simulink model "aaa"  (R2016b)
settings: Solver=ode4  StartTime=0.0  StopTime=inf  FixedStep=0.002  RelTol=1e-3  EnableMultiTasking=on
libraries: slrtlib x3
(part 3 of 5)

== stateflow chart aaa/Subsystem1/zidong/1#3 ==
  state zidong
    state chushihua
      entry:
      skhx=0;
      kghx=0;
      kgzhiling1=0;
      kgzhiling2=0;
      yjhx=0;
      gghx=0;
      ggzhiling1=0;
      ggzhiling2=0;
      skt=0;
      kgt=0;
      sdt=0;
      jst=0;
      ggt=0;
      yjt=0;
      skyichang=0;
      kgyichang=0;
      sdyichang=0;
      jsyichang=0;
      ggyichang=0;
      yjyichang=0;
    state on1
      entry:
      skhx=1;
    state songkaishijian
      entry:
      skt=skt+0.002;
    state start
      entry:
      yikaicishu = 0;
    state on10
      entry:
      skyichang=1;
    state songkaishijian1
      entry:
      skt=skt+0.002;
    state on8
      entry:
      skhx=0;
    state yanchishijian1
      entry:
      t=t+1;
    state tguiling
      entry: t=0;
    state on2
      entry:
      skhx=0;
      kghx=1;
      kgzhiling1=1;
      kgzhiling2=1;
    state kaigaishijian
      entry:
      kgt=kgt+0.002;
    state stop
      entry:
      skhx=0;
      kghx=0;
      kgzhiling1=0;
      kgzhiling2=0;
      yjhx=0;
      gghx=0;
      ggzhiling1=0;
      ggzhiling2=0;
      skt=0;
      kgt=0;
      sdt=0;
      jst=0;
      ggt=0;
      yjt=0;
    state songkaishijian2
      entry:
      kgt=kgt+0.002;
    state on9
      entry:
      kghx=0;
      kgzhiling1=0;
      kgzhiling2=0;
    state on11
      entry:
      kgyichang=1;
    state yanchishijian2
      entry:
      t2=t2+1;
    state t2guiling
      entry: t2=0;
    state on3
      entry:
      kghx=0;
      kgzhiling1=0;
      kgzhiling2=0;
      yjhx=1;
    state suodingshijian
      entry:
      sdt=sdt+0.002;
    state on7
      entry:
      yikaicishu = yikaicishu + 1;
    state songkaishijian3
      entry:
      sdt=sdt+0.002;
    state on13
      entry:
      yjhx=0;
    state on12
      entry:
      sdyichang=1;
    state yanchishijian3
      entry:
      t4=t4+1;
    state t4guiling
      entry: t4=0;
    state off
      entry:
      skhx=0;
      kghx=0;
      kgzhiling1=0;
      kgzhiling2=0;
      yjhx=0;
      gghx=0;
      ggzhiling1=0;
      ggzhiling2=0;
      skt=0;
      kgt=0;
      sdt=0;
      jst=0;
      ggt=0;
      yjt=0;
    state on4
      entry:
      yjhx=0;
      skhx=1;
    state jiesuoshijian
      entry:
      jst=jst+0.002;
    state songkaishijian4
      entry:
      jst=jst+0.002;
    state on15
      entry:
      skhx=0;
    state on14
      entry:
      jsyichang=1;
    state yanchishijian4
      entry:
      t6=t6+1;
    state t6guiling
      entry: t6=0;
    state on5
      entry:
      skhx=0;
      gghx=1;
      ggzhiling1=1;
      ggzhiling2=1;
    state guangaishijian
      entry:
      ggt=ggt+0.002;
    state songkaishijian5
      entry:
      ggt=ggt+0.002;
    state on17
      entry:
      gghx=0;
      ggzhiling1=0;
      ggzhiling2=0;
    state on16
      entry:
      ggyichang=1;
    state yanchishijian5
      entry:
      t8=t8+1;
    state t8guiling
      entry: t8=0;
    state yanchishijian6
      entry:
      t10=t10+1;
    state t10guiling
      entry: t10=0;
    state on6
      entry:
      gghx=0;
      ggzhiling1=0;
      ggzhiling2=0;
      yjhx=1;
    state yajinshijian
      entry:
      yjt=yjt+0.002;
    state songkaishijian6
      entry:
      yjt=yjt+0.002;
    state on19
      entry:
      yjhx=0;
    state on18
      entry:
      ggyichang=1;
    (default) -> start
    songkaishijian1 -> songkaishijian1 [order 1] : [jsdw==0||skdw==0]
    chushihua -> on1 : [start==1&&ggdw1==1&&ggdw2==1&&yjdw==1&&sddw==1]
    on1 -> (junction 48)
    (junction 48) -> songkaishijian [order 1] : [jsdw==0||skdw==0]
    start -> chushihua : [start==1]
    (junction 348) -> (junction 48) [order 1] : [skt<=2]
    (junction 48) -> tguiling [order 2] : [jsdw==1&&skdw==1]
    songkaishijian -> (junction 348)
    songkaishijian1 -> on8 [order 2] : [jsdw==1&&skdw==1]
    on10 -> songkaishijian1
    (junction 348) -> on10 [order 2] : [skt>2]
    (junction 54) -> yanchishijian1 [order 1] : [t<t1]
    yanchishijian1 -> (junction 54) : after(500,tick)
    tguiling -> (junction 54)
    (junction 54) -> on2 [order 2] : [t>=t1]
    (junction 190) -> chushihua [order 1] : [yikaicishu<shedingcishu&&jieshu==0]
    songkaishijian2 -> songkaishijian2 [order 1] : [kgdw1==0||kgdw2==0||jsdw==0||skdw==0]
    on2 -> (junction 65)
    (junction 65) -> kaigaishijian [order 1] : [kgdw1==0||kgdw2==0||jsdw==0||skdw==0]
    (junction 361) -> (junction 65) [order 2] : [kgt<=12]
    (junction 65) -> t2guiling [order 2] : [kgdw1==1&&kgdw2==1&&jsdw==1&&skdw==1]
    kaigaishijian -> (junction 361)
    (junction 76) -> yanchishijian2 [order 1] : [t2<t3]
    songkaishijian2 -> on9 [order 2] : [kgdw1==1&&kgdw2==1&&jsdw==1&&skdw==1]
    on11 -> songkaishijian2
    (junction 361) -> on11 [order 1] : [kgt>12]
    (junction 190) -> stop [order 2] : [yikaicishu>=shedingcishu||jieshu==1]
    on7 -> (junction 190)
    yanchishijian2 -> (junction 76) : after(500,tick)
    t2guiling -> (junction 76)
    (junction 76) -> on3 [order 2] : [t2>=t3]
    songkaishijian3 -> songkaishijian3 [order 1] : [kgdw1==0||kgdw2==0||sddw==0||yjdw==0]
    on3 -> (junction 96)
    (junction 96) -> suodingshijian [order 1] : [kgdw1==0||kgdw2==0||sddw==0||yjdw==0]
    (junction 386) -> (junction 96) [order 2] : [sdt<=2]
    (junction 96) -> t4guiling [order 2] : [kgdw1==1&&kgdw2==1&&sddw==1&&yjdw==1]
    off -> on7
    suodingshijian -> (junction 386)
    (junction 105) -> yanchishijian3 [order 1] : [t4<t5]
    songkaishijian3 -> on13 [order 2] : [kgdw1==1&&kgdw2==1&&jsdw==1&&skdw==1]
    on12 -> songkaishijian3
    (junction 386) -> on12 [order 1] : [sdt>2]
    yanchishijian3 -> (junction 105) : after(500,tick)
    t4guiling -> (junction 105)
    (junction 105) -> on4 [order 2] : [t4>=t5]
    songkaishijian4 -> songkaishijian4 [order 1] : [kgdw1==0||kgdw2==0||jsdw==0||skdw==0]
    on4 -> (junction 115)
    (junction 115) -> jiesuoshijian [order 1] : [kgdw1==0||kgdw2==0||jsdw==0||skdw==0]
    (junction 390) -> (junction 115) [order 2] : [jst<=2]
    (junction 115) -> t6guiling [order 2] : [kgdw1==1&&kgdw2==1&&jsdw==1&&skdw==1]
    jiesuoshijian -> (junction 390)
    (junction 125) -> yanchishijian4 [order 1] : [t6<t7]
    songkaishijian4 -> on15 [order 2] : [kgdw1==1&&kgdw2==1&&jsdw==1&&skdw==1]
    on14 -> songkaishijian4
    (junction 390) -> on14 [order 1] : [jst>2]
    yanchishijian4 -> (junction 125) : after(500,tick)
    t6guiling -> (junction 125)
    (junction 125) -> on5 [order 2] : [t6>=t7]
    (junction 339) -> off [order 2] : [t10>=t11]
    songkaishijian5 -> songkaishijian5 [order 2] : [ggdw1==0||ggdw2==0||jsdw==0||skdw==0]
    on5 -> (junction 142)
    (junction 142) -> guangaishijian [order 1] : [ggdw1==0||ggdw2==0||jsdw==0||skdw==0]
    (junction 403) -> (junction 142) [order 2] : [ggt<=12]
    (junction 142) -> t8guiling [order 2] : [ggdw1==1&&ggdw2==1&&jsdw==1&&skdw==1]
    guangaishijian -> (junction 403)
    (junction 154) -> yanchishijian5 [order 1] : [t8<t9]
    songkaishijian5 -> on17 [order 1] : [ggdw1==1&&ggdw2==1&&jsdw==1&&skdw==1]
    on16 -> songkaishijian5
    (junction 403) -> on16 [order 1] : [ggt>12]
    yanchishijian5 -> (junction 154) : after(500,tick)
    t8guiling -> (junction 154)
    (junction 154) -> on6 [order 2] : [t8>=t9]
    yanchishijian6 -> (junction 339) : after(500,tick)
    (junction 339) -> yanchishijian6 [order 1] : [t10<t11]
    t10guiling -> (junction 339)
    (junction 162) -> t10guiling [order 2] : [sddw==1&&yjdw==1&&ggdw1==1&&ggdw2==1]
    on6 -> (junction 162)
    (junction 162) -> yajinshijian [order 1] : [sddw==0||yjdw==0]
    songkaishijian6 -> songkaishijian6 [order 2] : [sddw==0||yjdw==0]
    (junction 410) -> (junction 162) [order 2] : [yjt<=2]
    yajinshijian -> (junction 410)
    songkaishijian6 -> on19 [order 1] : [sddw==1&&yjdw==1&&ggdw1==1&&ggdw2==1]
    on18 -> songkaishijian6
    (junction 410) -> on18 [order 1] : [yjt>2]
  (default) -> zidong
  data: start input; kgdw1 input; kgdw2 input; skhx output; kghx output; kgzhiling1 output; kgzhiling2 output; yjhx output; gghx output; ggzhiling1 output; ggzhiling2 output; skt output; kgt output; sdt output; jst output; ggt output; yjt output; ggdw1 input; ggdw2 input; kghc input; gghc input; sddw input; yjdw input; skdw input; jsdw input; t1 input; t3 input; t5 input; t7 input; t9 input; t11 input; t local; t2 local; t4 local; t6 local; t8 local; shedingcishu input; yikaicishu output; skyichang output; kgyichang output; sdyichang output; jsyichang output; jieshu input; t10 local; ggyichang output; yjyichang output

== stateflow chart aaa/Subsystem1/zidong/1#4 ==
  state zidong
    state chushihua
      entry:
      skhx=0;
      kghx=0;
      kgzhiling1=0;
      kgzhiling2=0;
      yjhx=0;
      gghx=0;
      ggzhiling1=0;
      ggzhiling2=0;
      skt=0;
      kgt=0;
      sdt=0;
      jst=0;
      ggt=0;
      yjt=0;
      skyichang=0;
      kgyichang=0;
      sdyichang=0;
      jsyichang=0;
      ggyichang=0;
      yjyichang=0;
    state on1
      entry:
      skhx=1;
    state songkaishijian
      entry:
      skt=skt+0.002;
    state start
      entry:
      yikaicishu = 0;
    state on10
      entry:
      skyichang=1;
    state songkaishijian1
      entry:
      skt=skt+0.002;
    state on8
      entry:
      skhx=0;
    state yanchishijian1
      entry:
      t=t+1;
    state tguiling
      entry: t=0;
    state on2
      entry:
      skhx=0;
      kghx=1;
      kgzhiling1=1;
      kgzhiling2=1;
    state kaigaishijian
      entry:
      kgt=kgt+0.002;
    state stop
      entry:
      skhx=0;
      kghx=0;
      kgzhiling1=0;
      kgzhiling2=0;
      yjhx=0;
      gghx=0;
      ggzhiling1=0;
      ggzhiling2=0;
      skt=0;
      kgt=0;
      sdt=0;
      jst=0;
      ggt=0;
      yjt=0;
    state songkaishijian2
      entry:
      kgt=kgt+0.002;
    state on9
      entry:
      kghx=0;
      kgzhiling1=0;
      kgzhiling2=0;
    state on11
      entry:
      kgyichang=1;
    state yanchishijian2
      entry:
      t2=t2+1;
    state t2guiling
      entry: t2=0;
    state on3
      entry:
      kghx=0;
      kgzhiling1=0;
      kgzhiling2=0;
      yjhx=1;
    state suodingshijian
      entry:
      sdt=sdt+0.002;
    state on7
      entry:
      yikaicishu = yikaicishu + 1;
    state songkaishijian3
      entry:
      sdt=sdt+0.002;
    state on13
      entry:
      yjhx=0;
    state on12
      entry:
      sdyichang=1;
    state yanchishijian3
      entry:
      t4=t4+1;
    state t4guiling
      entry: t4=0;
    state off
      entry:
      skhx=0;
      kghx=0;
      kgzhiling1=0;
      kgzhiling2=0;
      yjhx=0;
      gghx=0;
      ggzhiling1=0;
      ggzhiling2=0;
      skt=0;
      kgt=0;
      sdt=0;
      jst=0;
      ggt=0;
      yjt=0;
    state on4
      entry:
      yjhx=0;
      skhx=1;
    state jiesuoshijian
      entry:
      jst=jst+0.002;
    state songkaishijian4
      entry:
      jst=jst+0.002;
    state on15
      entry:
      skhx=0;
    state on14
      entry:
      jsyichang=1;
    state yanchishijian4
      entry:
      t6=t6+1;
    state t6guiling
      entry: t6=0;
    state on5
      entry:
      skhx=0;
      gghx=1;
      ggzhiling1=1;
      ggzhiling2=1;
    state guangaishijian
      entry:
      ggt=ggt+0.002;
    state songkaishijian5
      entry:
      ggt=ggt+0.002;
    state on17
      entry:
      gghx=0;
      ggzhiling1=0;
      ggzhiling2=0;
    state on16
      entry:
      ggyichang=1;
    state yanchishijian5
      entry:
      t8=t8+1;
    state t8guiling
      entry: t8=0;
    state yanchishijian6
      entry:
      t10=t10+1;
    state t10guiling
      entry: t10=0;
    state on6
      entry:
      gghx=0;
      ggzhiling1=0;
      ggzhiling2=0;
      yjhx=1;
    state yajinshijian
      entry:
      yjt=yjt+0.002;
    state songkaishijian6
      entry:
      yjt=yjt+0.002;
    state on19
      entry:
      yjhx=0;
    state on18
      entry:
      ggyichang=1;
    (default) -> start
    songkaishijian1 -> songkaishijian1 [order 1] : [jsdw==0||skdw==0]
    chushihua -> on1 : [start==1&&ggdw1==1&&ggdw2==1&&yjdw==1&&sddw==1]
    on1 -> (junction 48)
    (junction 48) -> songkaishijian [order 1] : [jsdw==0||skdw==0]
    start -> chushihua : [start==1]
    (junction 348) -> (junction 48) [order 1] : [skt<=2]
    (junction 48) -> tguiling [order 2] : [jsdw==1&&skdw==1]
    songkaishijian -> (junction 348)
    songkaishijian1 -> on8 [order 2] : [jsdw==1&&skdw==1]
    on10 -> songkaishijian1
    (junction 348) -> on10 [order 2] : [skt>2]
    (junction 54) -> yanchishijian1 [order 1] : [t<t1]
    yanchishijian1 -> (junction 54) : after(500,tick)
    tguiling -> (junction 54)
    (junction 54) -> on2 [order 2] : [t>=t1]
    (junction 190) -> chushihua [order 1] : [yikaicishu<shedingcishu&&jieshu==0]
    songkaishijian2 -> songkaishijian2 [order 1] : [kgdw1==0||kgdw2==0||jsdw==0||skdw==0]
    on2 -> (junction 65)
    (junction 65) -> kaigaishijian [order 1] : [kgdw1==0||kgdw2==0||jsdw==0||skdw==0]
    (junction 361) -> (junction 65) [order 2] : [kgt<=12]
    (junction 65) -> t2guiling [order 2] : [kgdw1==1&&kgdw2==1&&jsdw==1&&skdw==1]
    kaigaishijian -> (junction 361)
    (junction 76) -> yanchishijian2 [order 1] : [t2<t3]
    songkaishijian2 -> on9 [order 2] : [kgdw1==1&&kgdw2==1&&jsdw==1&&skdw==1]
    on11 -> songkaishijian2
    (junction 361) -> on11 [order 1] : [kgt>12]
    (junction 190) -> stop [order 2] : [yikaicishu>=shedingcishu||jieshu==1]
    on7 -> (junction 190)
    yanchishijian2 -> (junction 76) : after(500,tick)
    t2guiling -> (junction 76)
    (junction 76) -> on3 [order 2] : [t2>=t3]
    songkaishijian3 -> songkaishijian3 [order 1] : [kgdw1==0||kgdw2==0||sddw==0||yjdw==0]
    on3 -> (junction 96)
    (junction 96) -> suodingshijian [order 1] : [kgdw1==0||kgdw2==0||sddw==0||yjdw==0]
    (junction 386) -> (junction 96) [order 2] : [sdt<=2]
    (junction 96) -> t4guiling [order 2] : [kgdw1==1&&kgdw2==1&&sddw==1&&yjdw==1]
    off -> on7
    suodingshijian -> (junction 386)
    (junction 105) -> yanchishijian3 [order 1] : [t4<t5]
    songkaishijian3 -> on13 [order 2] : [kgdw1==1&&kgdw2==1&&jsdw==1&&skdw==1]
    on12 -> songkaishijian3
    (junction 386) -> on12 [order 1] : [sdt>2]
    yanchishijian3 -> (junction 105) : after(500,tick)
    t4guiling -> (junction 105)
    (junction 105) -> on4 [order 2] : [t4>=t5]
    songkaishijian4 -> songkaishijian4 [order 1] : [kgdw1==0||kgdw2==0||jsdw==0||skdw==0]
    on4 -> (junction 115)
    (junction 115) -> jiesuoshijian [order 1] : [kgdw1==0||kgdw2==0||jsdw==0||skdw==0]
    (junction 390) -> (junction 115) [order 2] : [jst<=2]
    (junction 115) -> t6guiling [order 2] : [kgdw1==1&&kgdw2==1&&jsdw==1&&skdw==1]
    jiesuoshijian -> (junction 390)
    (junction 125) -> yanchishijian4 [order 1] : [t6<t7]
    songkaishijian4 -> on15 [order 2] : [kgdw1==1&&kgdw2==1&&jsdw==1&&skdw==1]
    on14 -> songkaishijian4
    (junction 390) -> on14 [order 1] : [jst>2]
    yanchishijian4 -> (junction 125) : after(500,tick)
    t6guiling -> (junction 125)
    (junction 125) -> on5 [order 2] : [t6>=t7]
    (junction 339) -> off [order 2] : [t10>=t11]
    songkaishijian5 -> songkaishijian5 [order 2] : [ggdw1==0||ggdw2==0||jsdw==0||skdw==0]
    on5 -> (junction 142)
    (junction 142) -> guangaishijian [order 1] : [ggdw1==0||ggdw2==0||jsdw==0||skdw==0]
    (junction 403) -> (junction 142) [order 2] : [ggt<=12]
    (junction 142) -> t8guiling [order 2] : [ggdw1==1&&ggdw2==1&&jsdw==1&&skdw==1]
    guangaishijian -> (junction 403)
    (junction 154) -> yanchishijian5 [order 1] : [t8<t9]
    songkaishijian5 -> on17 [order 1] : [ggdw1==1&&ggdw2==1&&jsdw==1&&skdw==1]
    on16 -> songkaishijian5
    (junction 403) -> on16 [order 1] : [ggt>12]
    yanchishijian5 -> (junction 154) : after(500,tick)
    t8guiling -> (junction 154)
    (junction 154) -> on6 [order 2] : [t8>=t9]
    yanchishijian6 -> (junction 339) : after(500,tick)
    (junction 339) -> yanchishijian6 [order 1] : [t10<t11]
    t10guiling -> (junction 339)
    (junction 162) -> t10guiling [order 2] : [sddw==1&&yjdw==1&&ggdw1==1&&ggdw2==1]
    on6 -> (junction 162)
    (junction 162) -> yajinshijian [order 1] : [sddw==0||yjdw==0]
    songkaishijian6 -> songkaishijian6 [order 2] : [sddw==0||yjdw==0]
    (junction 410) -> (junction 162) [order 2] : [yjt<=2]
    yajinshijian -> (junction 410)
    songkaishijian6 -> on19 [order 1] : [sddw==1&&yjdw==1&&ggdw1==1&&ggdw2==1]
    on18 -> songkaishijian6
    (junction 410) -> on18 [order 1] : [yjt>2]
  (default) -> zidong
  data: start input; kgdw1 input; kgdw2 input; skhx output; kghx output; kgzhiling1 output; kgzhiling2 output; yjhx output; gghx output; ggzhiling1 output; ggzhiling2 output; skt output; kgt output; sdt output; jst output; ggt output; yjt output; ggdw1 input; ggdw2 input; kghc input; gghc input; sddw input; yjdw input; skdw input; jsdw input; t1 input; t3 input; t5 input; t7 input; t9 input; t11 input; t local; t2 local; t4 local; t6 local; t8 local; shedingcishu input; yikaicishu output; skyichang output; kgyichang output; sdyichang output; jsyichang output; jieshu input; t10 local; ggyichang output; yjyichang output

== stateflow chart aaa/Subsystem1/zidong/1#5 ==
  state zidong
    state chushihua
      entry:
      skhx=0;
      kghx=0;
      kgzhiling1=0;
      kgzhiling2=0;
      yjhx=0;
      gghx=0;
      ggzhiling1=0;
      ggzhiling2=0;
      skt=0;
      kgt=0;
      sdt=0;
      jst=0;
      ggt=0;
      yjt=0;
      skyichang=0;
      kgyichang=0;
      sdyichang=0;
      jsyichang=0;
      ggyichang=0;
      yjyichang=0;
    state on1
      entry:
      skhx=1;
    state songkaishijian
      entry:
      skt=skt+0.002;
    state start
      entry:
      yikaicishu = 0;
    state on10
      entry:
      skyichang=1;
    state songkaishijian1
      entry:
      skt=skt+0.002;
    state on8
      entry:
      skhx=0;
    state yanchishijian1
      entry:
      t=t+1;
    state tguiling
      entry: t=0;
    state on2
      entry:
      skhx=0;
      kghx=1;
      kgzhiling1=1;
      kgzhiling2=1;
    state kaigaishijian
      entry:
      kgt=kgt+0.002;
    state stop
      entry:
      skhx=0;
      kghx=0;
      kgzhiling1=0;
      kgzhiling2=0;
      yjhx=0;
      gghx=0;
      ggzhiling1=0;
      ggzhiling2=0;
      skt=0;
      kgt=0;
      sdt=0;
      jst=0;
      ggt=0;
      yjt=0;
    state songkaishijian2
      entry:
      kgt=kgt+0.002;
    state on9
      entry:
      kghx=0;
      kgzhiling1=0;
      kgzhiling2=0;
    state on11
      entry:
      kgyichang=1;
    state yanchishijian2
      entry:
      t2=t2+1;
    state t2guiling
      entry: t2=0;
    state on3
      entry:
      kghx=0;
      kgzhiling1=0;
      kgzhiling2=0;
      yjhx=1;
    state suodingshijian
      entry:
      sdt=sdt+0.002;
    state on7
      entry:
      yikaicishu = yikaicishu + 1;
    state songkaishijian3
      entry:
      sdt=sdt+0.002;
    state on13
      entry:
      yjhx=0;
    state on12
      entry:
      sdyichang=1;
    state yanchishijian3
      entry:
      t4=t4+1;
    state t4guiling
      entry: t4=0;
    state off
      entry:
      skhx=0;
      kghx=0;
      kgzhiling1=0;
      kgzhiling2=0;
      yjhx=0;
      gghx=0;
      ggzhiling1=0;
      ggzhiling2=0;
      skt=0;
      kgt=0;
      sdt=0;
      jst=0;
      ggt=0;
      yjt=0;
    state on4
      entry:
      yjhx=0;
      skhx=1;
    state jiesuoshijian
      entry:
      jst=jst+0.002;
    state songkaishijian4
      entry:
      jst=jst+0.002;
    state on15
      entry:
      skhx=0;
    state on14
      entry:
      jsyichang=1;
    state yanchishijian4
      entry:
      t6=t6+1;
    state t6guiling
      entry: t6=0;
    state on5
      entry:
      skhx=0;
      gghx=1;
      ggzhiling1=1;
      ggzhiling2=1;
    state guangaishijian
      entry:
      ggt=ggt+0.002;
    state songkaishijian5
      entry:
      ggt=ggt+0.002;
    state on17
      entry:
      gghx=0;
      ggzhiling1=0;
      ggzhiling2=0;
    state on16
      entry:
      ggyichang=1;
    state yanchishijian5
      entry:
      t8=t8+1;
    state t8guiling
      entry: t8=0;
    state yanchishijian6
      entry:
      t10=t10+1;
    state t10guiling
      entry: t10=0;
    state on6
      entry:
      gghx=0;
      ggzhiling1=0;
      ggzhiling2=0;
      yjhx=1;
    state yajinshijian
      entry:
      yjt=yjt+0.002;
    state songkaishijian6
      entry:
      yjt=yjt+0.002;
    state on19
      entry:
      yjhx=0;
    state on18
      entry:
      ggyichang=1;
    (default) -> start
    songkaishijian1 -> songkaishijian1 [order 1] : [jsdw==0||skdw==0]
    chushihua -> on1 : [start==1&&ggdw1==1&&ggdw2==1&&yjdw==1&&sddw==1]
    on1 -> (junction 48)
    (junction 48) -> songkaishijian [order 1] : [jsdw==0||skdw==0]
    start -> chushihua : [start==1]
    (junction 348) -> (junction 48) [order 1] : [skt<=2]
    (junction 48) -> tguiling [order 2] : [jsdw==1&&skdw==1]
    songkaishijian -> (junction 348)
    songkaishijian1 -> on8 [order 2] : [jsdw==1&&skdw==1]
    on10 -> songkaishijian1
    (junction 348) -> on10 [order 2] : [skt>2]
    (junction 54) -> yanchishijian1 [order 1] : [t<t1]
    yanchishijian1 -> (junction 54) : after(500,tick)
    tguiling -> (junction 54)
    (junction 54) -> on2 [order 2] : [t>=t1]
    (junction 190) -> chushihua [order 1] : [yikaicishu<shedingcishu&&jieshu==0]
    songkaishijian2 -> songkaishijian2 [order 1] : [kgdw1==0||kgdw2==0||jsdw==0||skdw==0]
    on2 -> (junction 65)
    (junction 65) -> kaigaishijian [order 1] : [kgdw1==0||kgdw2==0||jsdw==0||skdw==0]
    (junction 361) -> (junction 65) [order 2] : [kgt<=12]
    (junction 65) -> t2guiling [order 2] : [kgdw1==1&&kgdw2==1&&jsdw==1&&skdw==1]
    kaigaishijian -> (junction 361)
    (junction 76) -> yanchishijian2 [order 1] : [t2<t3]
    songkaishijian2 -> on9 [order 2] : [kgdw1==1&&kgdw2==1&&jsdw==1&&skdw==1]
    on11 -> songkaishijian2
    (junction 361) -> on11 [order 1] : [kgt>12]
    (junction 190) -> stop [order 2] : [yikaicishu>=shedingcishu||jieshu==1]
    on7 -> (junction 190)
    yanchishijian2 -> (junction 76) : after(500,tick)
    t2guiling -> (junction 76)
    (junction 76) -> on3 [order 2] : [t2>=t3]
    songkaishijian3 -> songkaishijian3 [order 1] : [kgdw1==0||kgdw2==0||sddw==0||yjdw==0]
    on3 -> (junction 96)
    (junction 96) -> suodingshijian [order 1] : [kgdw1==0||kgdw2==0||sddw==0||yjdw==0]
    (junction 386) -> (junction 96) [order 2] : [sdt<=2]
    (junction 96) -> t4guiling [order 2] : [kgdw1==1&&kgdw2==1&&sddw==1&&yjdw==1]
    off -> on7
    suodingshijian -> (junction 386)
    (junction 105) -> yanchishijian3 [order 1] : [t4<t5]
    songkaishijian3 -> on13 [order 2] : [kgdw1==1&&kgdw2==1&&jsdw==1&&skdw==1]
    on12 -> songkaishijian3
    (junction 386) -> on12 [order 1] : [sdt>2]
    yanchishijian3 -> (junction 105) : after(500,tick)
    t4guiling -> (junction 105)
    (junction 105) -> on4 [order 2] : [t4>=t5]
    songkaishijian4 -> songkaishijian4 [order 1] : [kgdw1==0||kgdw2==0||jsdw==0||skdw==0]
    on4 -> (junction 115)
    (junction 115) -> jiesuoshijian [order 1] : [kgdw1==0||kgdw2==0||jsdw==0||skdw==0]
    (junction 390) -> (junction 115) [order 2] : [jst<=2]
    (junction 115) -> t6guiling [order 2] : [kgdw1==1&&kgdw2==1&&jsdw==1&&skdw==1]
    jiesuoshijian -> (junction 390)
    (junction 125) -> yanchishijian4 [order 1] : [t6<t7]
    songkaishijian4 -> on15 [order 2] : [kgdw1==1&&kgdw2==1&&jsdw==1&&skdw==1]
    on14 -> songkaishijian4
    (junction 390) -> on14 [order 1] : [jst>2]
    yanchishijian4 -> (junction 125) : after(500,tick)
    t6guiling -> (junction 125)
    (junction 125) -> on5 [order 2] : [t6>=t7]
    (junction 339) -> off [order 2] : [t10>=t11]
    songkaishijian5 -> songkaishijian5 [order 2] : [ggdw1==0||ggdw2==0||jsdw==0||skdw==0]
    on5 -> (junction 142)
    (junction 142) -> guangaishijian [order 1] : [ggdw1==0||ggdw2==0||jsdw==0||skdw==0]
    (junction 403) -> (junction 142) [order 2] : [ggt<=12]
    (junction 142) -> t8guiling [order 2] : [ggdw1==1&&ggdw2==1&&jsdw==1&&skdw==1]
    guangaishijian -> (junction 403)
    (junction 154) -> yanchishijian5 [order 1] : [t8<t9]
    songkaishijian5 -> on17 [order 1] : [ggdw1==1&&ggdw2==1&&jsdw==1&&skdw==1]
    on16 -> songkaishijian5
    (junction 403) -> on16 [order 1] : [ggt>12]
    yanchishijian5 -> (junction 154) : after(500,tick)
    t8guiling -> (junction 154)
    (junction 154) -> on6 [order 2] : [t8>=t9]
    yanchishijian6 -> (junction 339) : after(500,tick)
    (junction 339) -> yanchishijian6 [order 1] : [t10<t11]
    t10guiling -> (junction 339)
    (junction 162) -> t10guiling [order 2] : [sddw==1&&yjdw==1&&ggdw1==1&&ggdw2==1]
    on6 -> (junction 162)
    (junction 162) -> yajinshijian [order 1] : [sddw==0||yjdw==0]
    songkaishijian6 -> songkaishijian6 [order 2] : [sddw==0||yjdw==0]
    (junction 410) -> (junction 162) [order 2] : [yjt<=2]
    yajinshijian -> (junction 410)
    songkaishijian6 -> on19 [order 1] : [sddw==1&&yjdw==1&&ggdw1==1&&ggdw2==1]
    on18 -> songkaishijian6
    (junction 410) -> on18 [order 1] : [yjt>2]
  (default) -> zidong
  data: start input; kgdw1 input; kgdw2 input; skhx output; kghx output; kgzhiling1 output; kgzhiling2 output; yjhx output; gghx output; ggzhiling1 output; ggzhiling2 output; skt output; kgt output; sdt output; jst output; ggt output; yjt output; ggdw1 input; ggdw2 input; kghc input; gghc input; sddw input; yjdw input; skdw input; jsdw input; t1 input; t3 input; t5 input; t7 input; t9 input; t11 input; t local; t2 local; t4 local; t6 local; t8 local; shedingcishu input; yikaicishu output; skyichang output; kgyichang output; sdyichang output; jsyichang output; jieshu input; t10 local; ggyichang output; yjyichang output

== stateflow chart aaa/Subsystem1/zidong/1#6 ==
  state zidong
    state chushihua
      entry:
      skhx=0;
      kghx=0;
      kgzhiling1=0;
      kgzhiling2=0;
      yjhx=0;
      gghx=0;
      ggzhiling1=0;
      ggzhiling2=0;
      skt=0;
      kgt=0;
      sdt=0;
      jst=0;
      ggt=0;
      yjt=0;
      skyichang=0;
      kgyichang=0;
      sdyichang=0;
      jsyichang=0;
      ggyichang=0;
      yjyichang=0;
    state on1
      entry:
      skhx=1;
    state songkaishijian
      entry:
      skt=skt+0.002;
    state start
      entry:
      yikaicishu = 0;
    state on10
      entry:
      skyichang=1;
    state songkaishijian1
      entry:
      skt=skt+0.002;
    state on8
      entry:
      skhx=0;
    state yanchishijian1
      entry:
      t=t+1;
    state tguiling
      entry: t=0;
    state on2
      entry:
      skhx=0;
      kghx=1;
      kgzhiling1=1;
      kgzhiling2=1;
    state kaigaishijian
      entry:
      kgt=kgt+0.002;
    state stop
      entry:
      skhx=0;
      kghx=0;
      kgzhiling1=0;
      kgzhiling2=0;
      yjhx=0;
      gghx=0;
      ggzhiling1=0;
      ggzhiling2=0;
      skt=0;
      kgt=0;
      sdt=0;
      jst=0;
      ggt=0;
      yjt=0;
    state songkaishijian2
      entry:
      kgt=kgt+0.002;
    state on9
      entry:
      kghx=0;
      kgzhiling1=0;
      kgzhiling2=0;
    state on11
      entry:
      kgyichang=1;
    state yanchishijian2
      entry:
      t2=t2+1;
    state t2guiling
      entry: t2=0;
    state on3
      entry:
      kghx=0;
      kgzhiling1=0;
      kgzhiling2=0;
      yjhx=1;
    state suodingshijian
      entry:
      sdt=sdt+0.002;
    state on7
      entry:
      yikaicishu = yikaicishu + 1;
    state songkaishijian3
      entry:
      sdt=sdt+0.002;
    state on13
      entry:
      yjhx=0;
    state on12
      entry:
      sdyichang=1;
    state yanchishijian3
      entry:
      t4=t4+1;
    state t4guiling
      entry: t4=0;
    state off
      entry:
      skhx=0;
      kghx=0;
      kgzhiling1=0;
      kgzhiling2=0;
      yjhx=0;
      gghx=0;
      ggzhiling1=0;
      ggzhiling2=0;
      skt=0;
      kgt=0;
      sdt=0;
      jst=0;
      ggt=0;
      yjt=0;
    state on4
      entry:
      yjhx=0;
      skhx=1;
    state jiesuoshijian
      entry:
      jst=jst+0.002;
    state songkaishijian4
      entry:
      jst=jst+0.002;
    state on15
      entry:
      skhx=0;
    state on14
      entry:
      jsyichang=1;
    state yanchishijian4
      entry:
      t6=t6+1;
    state t6guiling
      entry: t6=0;
    state on5
      entry:
      skhx=0;
      gghx=1;
      ggzhiling1=1;
      ggzhiling2=1;
    state guangaishijian
      entry:
      ggt=ggt+0.002;
    state songkaishijian5
      entry:
      ggt=ggt+0.002;
    state on17
      entry:
      gghx=0;
      ggzhiling1=0;
      ggzhiling2=0;
    state on16
      entry:
      ggyichang=1;
    state yanchishijian5
      entry:
      t8=t8+1;
    state t8guiling
      entry: t8=0;
    state yanchishijian6
      entry:
      t10=t10+1;
    state t10guiling
      entry: t10=0;
    state on6
      entry:
      gghx=0;
      ggzhiling1=0;
      ggzhiling2=0;
      yjhx=1;
    state yajinshijian
      entry:
      yjt=yjt+0.002;
    state songkaishijian6
      entry:
      yjt=yjt+0.002;
    state on19
      entry:
      yjhx=0;
    state on18
      entry:
      ggyichang=1;
    (default) -> start
    songkaishijian1 -> songkaishijian1 [order 1] : [jsdw==0||skdw==0]
    chushihua -> on1 : [start==1&&ggdw1==1&&ggdw2==1&&yjdw==1&&sddw==1]
    on1 -> (junction 48)
    (junction 48) -> songkaishijian [order 1] : [jsdw==0||skdw==0]
    start -> chushihua : [start==1]
    (junction 348) -> (junction 48) [order 1] : [skt<=2]
    (junction 48) -> tguiling [order 2] : [jsdw==1&&skdw==1]
    songkaishijian -> (junction 348)
    songkaishijian1 -> on8 [order 2] : [jsdw==1&&skdw==1]
    on10 -> songkaishijian1
    (junction 348) -> on10 [order 2] : [skt>2]
    (junction 54) -> yanchishijian1 [order 1] : [t<t1]
    yanchishijian1 -> (junction 54) : after(500,tick)
    tguiling -> (junction 54)
    (junction 54) -> on2 [order 2] : [t>=t1]
    (junction 190) -> chushihua [order 1] : [yikaicishu<shedingcishu&&jieshu==0]
    songkaishijian2 -> songkaishijian2 [order 1] : [kgdw1==0||kgdw2==0||jsdw==0||skdw==0]
    on2 -> (junction 65)
    (junction 65) -> kaigaishijian [order 1] : [kgdw1==0||kgdw2==0||jsdw==0||skdw==0]
    (junction 361) -> (junction 65) [order 2] : [kgt<=12]
    (junction 65) -> t2guiling [order 2] : [kgdw1==1&&kgdw2==1&&jsdw==1&&skdw==1]
    kaigaishijian -> (junction 361)
    (junction 76) -> yanchishijian2 [order 1] : [t2<t3]
    songkaishijian2 -> on9 [order 2] : [kgdw1==1&&kgdw2==1&&jsdw==1&&skdw==1]
    on11 -> songkaishijian2
    (junction 361) -> on11 [order 1] : [kgt>12]
    (junction 190) -> stop [order 2] : [yikaicishu>=shedingcishu||jieshu==1]
    on7 -> (junction 190)
    yanchishijian2 -> (junction 76) : after(500,tick)
    t2guiling -> (junction 76)
    (junction 76) -> on3 [order 2] : [t2>=t3]
    songkaishijian3 -> songkaishijian3 [order 1] : [kgdw1==0||kgdw2==0||sddw==0||yjdw==0]
    on3 -> (junction 96)
    (junction 96) -> suodingshijian [order 1] : [kgdw1==0||kgdw2==0||sddw==0||yjdw==0]
    (junction 386) -> (junction 96) [order 2] : [sdt<=2]
    (junction 96) -> t4guiling [order 2] : [kgdw1==1&&kgdw2==1&&sddw==1&&yjdw==1]
    off -> on7
    suodingshijian -> (junction 386)
    (junction 105) -> yanchishijian3 [order 1] : [t4<t5]
    songkaishijian3 -> on13 [order 2] : [kgdw1==1&&kgdw2==1&&jsdw==1&&skdw==1]
    on12 -> songkaishijian3
    (junction 386) -> on12 [order 1] : [sdt>2]
    yanchishijian3 -> (junction 105) : after(500,tick)
    t4guiling -> (junction 105)
    (junction 105) -> on4 [order 2] : [t4>=t5]
    songkaishijian4 -> songkaishijian4 [order 1] : [kgdw1==0||kgdw2==0||jsdw==0||skdw==0]
    on4 -> (junction 115)
    (junction 115) -> jiesuoshijian [order 1] : [kgdw1==0||kgdw2==0||jsdw==0||skdw==0]
    (junction 390) -> (junction 115) [order 2] : [jst<=2]
    (junction 115) -> t6guiling [order 2] : [kgdw1==1&&kgdw2==1&&jsdw==1&&skdw==1]
    jiesuoshijian -> (junction 390)
    (junction 125) -> yanchishijian4 [order 1] : [t6<t7]
    songkaishijian4 -> on15 [order 2] : [kgdw1==1&&kgdw2==1&&jsdw==1&&skdw==1]
    on14 -> songkaishijian4
    (junction 390) -> on14 [order 1] : [jst>2]
    yanchishijian4 -> (junction 125) : after(500,tick)
    t6guiling -> (junction 125)
    (junction 125) -> on5 [order 2] : [t6>=t7]
    (junction 339) -> off [order 2] : [t10>=t11]
    songkaishijian5 -> songkaishijian5 [order 2] : [ggdw1==0||ggdw2==0||jsdw==0||skdw==0]
    on5 -> (junction 142)
    (junction 142) -> guangaishijian [order 1] : [ggdw1==0||ggdw2==0||jsdw==0||skdw==0]
    (junction 403) -> (junction 142) [order 2] : [ggt<=12]
    (junction 142) -> t8guiling [order 2] : [ggdw1==1&&ggdw2==1&&jsdw==1&&skdw==1]
    guangaishijian -> (junction 403)
    (junction 154) -> yanchishijian5 [order 1] : [t8<t9]
    songkaishijian5 -> on17 [order 1] : [ggdw1==1&&ggdw2==1&&jsdw==1&&skdw==1]
    on16 -> songkaishijian5
    (junction 403) -> on16 [order 1] : [ggt>12]
    yanchishijian5 -> (junction 154) : after(500,tick)
    t8guiling -> (junction 154)
    (junction 154) -> on6 [order 2] : [t8>=t9]
    yanchishijian6 -> (junction 339) : after(500,tick)
    (junction 339) -> yanchishijian6 [order 1] : [t10<t11]
    t10guiling -> (junction 339)
    (junction 162) -> t10guiling [order 2] : [sddw==1&&yjdw==1&&ggdw1==1&&ggdw2==1]
    on6 -> (junction 162)
    (junction 162) -> yajinshijian [order 1] : [sddw==0||yjdw==0]
    songkaishijian6 -> songkaishijian6 [order 2] : [sddw==0||yjdw==0]
    (junction 410) -> (junction 162) [order 2] : [yjt<=2]
    yajinshijian -> (junction 410)
    songkaishijian6 -> on19 [order 1] : [sddw==1&&yjdw==1&&ggdw1==1&&ggdw2==1]
    on18 -> songkaishijian6
    (junction 410) -> on18 [order 1] : [yjt>2]
  (default) -> zidong
  data: start input; kgdw1 input; kgdw2 input; skhx output; kghx output; kgzhiling1 output; kgzhiling2 output; yjhx output; gghx output; ggzhiling1 output; ggzhiling2 output; skt output; kgt output; sdt output; jst output; ggt output; yjt output; ggdw1 input; ggdw2 input; kghc input; gghc input; sddw input; yjdw input; skdw input; jsdw input; t1 input; t3 input; t5 input; t7 input; t9 input; t11 input; t local; t2 local; t4 local; t6 local; t8 local; shedingcishu input; yikaicishu output; skyichang output; kgyichang output; sdyichang output; jsyichang output; jieshu input; t10 local; ggyichang output; yjyichang output

== stateflow chart aaa/Subsystem1/zidong/1#7 ==
  state zidong
    state chushihua
      entry:
      skhx=0;
      kghx=0;
      kgzhiling1=0;
      kgzhiling2=0;
      yjhx=0;
      gghx=0;
      ggzhiling1=0;
      ggzhiling2=0;
      skt=0;
      kgt=0;
      sdt=0;
      jst=0;
      ggt=0;
      yjt=0;
      skyichang=0;
      kgyichang=0;
      sdyichang=0;
      jsyichang=0;
      ggyichang=0;
      yjyichang=0;
    state on1
      entry:
      skhx=1;
    state songkaishijian
      entry:
      skt=skt+0.002;
    state start
      entry:
      yikaicishu = 0;
    state on10
      entry:
      skyichang=1;
    state songkaishijian1
      entry:
      skt=skt+0.002;
    state on8
      entry:
      skhx=0;
    state yanchishijian1
      entry:
      t=t+1;
    state tguiling
      entry: t=0;
    state on2
      entry:
      skhx=0;
      kghx=1;
      kgzhiling1=1;
      kgzhiling2=1;
    state kaigaishijian
      entry:
      kgt=kgt+0.002;
    state stop
      entry:
      skhx=0;
      kghx=0;
      kgzhiling1=0;
      kgzhiling2=0;
      yjhx=0;
      gghx=0;
      ggzhiling1=0;
      ggzhiling2=0;
      skt=0;
      kgt=0;
      sdt=0;
      jst=0;
      ggt=0;
      yjt=0;
    state songkaishijian2
      entry:
      kgt=kgt+0.002;
    state on9
      entry:
      kghx=0;
      kgzhiling1=0;
      kgzhiling2=0;
    state on11
      entry:
      kgyichang=1;
    state yanchishijian2
      entry:
      t2=t2+1;
    state t2guiling
      entry: t2=0;
    state on3
      entry:
      kghx=0;
      kgzhiling1=0;
      kgzhiling2=0;
      yjhx=1;
    state suodingshijian
      entry:
      sdt=sdt+0.002;
    state on7
      entry:
      yikaicishu = yikaicishu + 1;
    state songkaishijian3
      entry:
      sdt=sdt+0.002;
    state on13
      entry:
      yjhx=0;
    state on12
      entry:
      sdyichang=1;
    state yanchishijian3
      entry:
      t4=t4+1;
    state t4guiling
      entry: t4=0;
    state off
      entry:
      skhx=0;
      kghx=0;
      kgzhiling1=0;
      kgzhiling2=0;
      yjhx=0;
      gghx=0;
      ggzhiling1=0;
      ggzhiling2=0;
      skt=0;
      kgt=0;
      sdt=0;
      jst=0;
      ggt=0;
      yjt=0;
    state on4
      entry:
      yjhx=0;
      skhx=1;
    state jiesuoshijian
      entry:
      jst=jst+0.002;
    state songkaishijian4
      entry:
      jst=jst+0.002;
    state on15
      entry:
      skhx=0;
    state on14
      entry:
      jsyichang=1;
    state yanchishijian4
      entry:
      t6=t6+1;
    state t6guiling
      entry: t6=0;
    state on5
      entry:
      skhx=0;
      gghx=1;
      ggzhiling1=1;
      ggzhiling2=1;
    state guangaishijian
      entry:
      ggt=ggt+0.002;
    state songkaishijian5
      entry:
      ggt=ggt+0.002;
    state on17
      entry:
      gghx=0;
      ggzhiling1=0;
      ggzhiling2=0;
    state on16
      entry:
      ggyichang=1;
    state yanchishijian5
      entry:
      t8=t8+1;
    state t8guiling
      entry: t8=0;
    state yanchishijian6
      entry:
      t10=t10+1;
    state t10guiling
      entry: t10=0;
    state on6
      entry:
      gghx=0;
      ggzhiling1=0;
      ggzhiling2=0;
      yjhx=1;
    state yajinshijian
      entry:
      yjt=yjt+0.002;
    state songkaishijian6
      entry:
      yjt=yjt+0.002;
    state on19
      entry:
      yjhx=0;
    state on18
      entry:
      ggyichang=1;
    (default) -> start
    songkaishijian1 -> songkaishijian1 [order 1] : [jsdw==0||skdw==0]
    chushihua -> on1 : [start==1&&ggdw1==1&&ggdw2==1&&yjdw==1&&sddw==1]
    on1 -> (junction 48)
    (junction 48) -> songkaishijian [order 1] : [jsdw==0||skdw==0]
    start -> chushihua : [start==1]
    (junction 348) -> (junction 48) [order 1] : [skt<=2]
    (junction 48) -> tguiling [order 2] : [jsdw==1&&skdw==1]
    songkaishijian -> (junction 348)
    songkaishijian1 -> on8 [order 2] : [jsdw==1&&skdw==1]
    on10 -> songkaishijian1
    (junction 348) -> on10 [order 2] : [skt>2]
    (junction 54) -> yanchishijian1 [order 1] : [t<t1]
    yanchishijian1 -> (junction 54) : after(500,tick)
    tguiling -> (junction 54)
    (junction 54) -> on2 [order 2] : [t>=t1]
    (junction 190) -> chushihua [order 1] : [yikaicishu<shedingcishu&&jieshu==0]
    songkaishijian2 -> songkaishijian2 [order 1] : [kgdw1==0||kgdw2==0||jsdw==0||skdw==0]
    on2 -> (junction 65)
    (junction 65) -> kaigaishijian [order 1] : [kgdw1==0||kgdw2==0||jsdw==0||skdw==0]
    (junction 361) -> (junction 65) [order 2] : [kgt<=12]
    (junction 65) -> t2guiling [order 2] : [kgdw1==1&&kgdw2==1&&jsdw==1&&skdw==1]
    kaigaishijian -> (junction 361)
    (junction 76) -> yanchishijian2 [order 1] : [t2<t3]
    songkaishijian2 -> on9 [order 2] : [kgdw1==1&&kgdw2==1&&jsdw==1&&skdw==1]
    on11 -> songkaishijian2
    (junction 361) -> on11 [order 1] : [kgt>12]
    (junction 190) -> stop [order 2] : [yikaicishu>=shedingcishu||jieshu==1]
    on7 -> (junction 190)
    yanchishijian2 -> (junction 76) : after(500,tick)
    t2guiling -> (junction 76)
    (junction 76) -> on3 [order 2] : [t2>=t3]
    songkaishijian3 -> songkaishijian3 [order 1] : [kgdw1==0||kgdw2==0||sddw==0||yjdw==0]
    on3 -> (junction 96)
    (junction 96) -> suodingshijian [order 1] : [kgdw1==0||kgdw2==0||sddw==0||yjdw==0]
    (junction 386) -> (junction 96) [order 2] : [sdt<=2]
    (junction 96) -> t4guiling [order 2] : [kgdw1==1&&kgdw2==1&&sddw==1&&yjdw==1]
    off -> on7
    suodingshijian -> (junction 386)
    (junction 105) -> yanchishijian3 [order 1] : [t4<t5]
    songkaishijian3 -> on13 [order 2] : [kgdw1==1&&kgdw2==1&&jsdw==1&&skdw==1]
    on12 -> songkaishijian3
    (junction 386) -> on12 [order 1] : [sdt>2]
    yanchishijian3 -> (junction 105) : after(500,tick)
    t4guiling -> (junction 105)
    (junction 105) -> on4 [order 2] : [t4>=t5]
    songkaishijian4 -> songkaishijian4 [order 1] : [kgdw1==0||kgdw2==0||jsdw==0||skdw==0]
    on4 -> (junction 115)
    (junction 115) -> jiesuoshijian [order 1] : [kgdw1==0||kgdw2==0||jsdw==0||skdw==0]
    (junction 390) -> (junction 115) [order 2] : [jst<=2]
    (junction 115) -> t6guiling [order 2] : [kgdw1==1&&kgdw2==1&&jsdw==1&&skdw==1]
    jiesuoshijian -> (junction 390)
    (junction 125) -> yanchishijian4 [order 1] : [t6<t7]
    songkaishijian4 -> on15 [order 2] : [kgdw1==1&&kgdw2==1&&jsdw==1&&skdw==1]
    on14 -> songkaishijian4
    (junction 390) -> on14 [order 1] : [jst>2]
    yanchishijian4 -> (junction 125) : after(500,tick)
    t6guiling -> (junction 125)
    (junction 125) -> on5 [order 2] : [t6>=t7]
    (junction 339) -> off [order 2] : [t10>=t11]
    songkaishijian5 -> songkaishijian5 [order 2] : [ggdw1==0||ggdw2==0||jsdw==0||skdw==0]
    on5 -> (junction 142)
    (junction 142) -> guangaishijian [order 1] : [ggdw1==0||ggdw2==0||jsdw==0||skdw==0]
    (junction 403) -> (junction 142) [order 2] : [ggt<=12]
    (junction 142) -> t8guiling [order 2] : [ggdw1==1&&ggdw2==1&&jsdw==1&&skdw==1]
    guangaishijian -> (junction 403)
    (junction 154) -> yanchishijian5 [order 1] : [t8<t9]
    songkaishijian5 -> on17 [order 1] : [ggdw1==1&&ggdw2==1&&jsdw==1&&skdw==1]
    on16 -> songkaishijian5
    (junction 403) -> on16 [order 1] : [ggt>12]
    yanchishijian5 -> (junction 154) : after(500,tick)
    t8guiling -> (junction 154)
    (junction 154) -> on6 [order 2] : [t8>=t9]
    yanchishijian6 -> (junction 339) : after(500,tick)
    (junction 339) -> yanchishijian6 [order 1] : [t10<t11]
    t10guiling -> (junction 339)
    (junction 162) -> t10guiling [order 2] : [sddw==1&&yjdw==1&&ggdw1==1&&ggdw2==1]
    on6 -> (junction 162)
    (junction 162) -> yajinshijian [order 1] : [sddw==0||yjdw==0]
    songkaishijian6 -> songkaishijian6 [order 2] : [sddw==0||yjdw==0]
    (junction 410) -> (junction 162) [order 2] : [yjt<=2]
    yajinshijian -> (junction 410)
    songkaishijian6 -> on19 [order 1] : [sddw==1&&yjdw==1&&ggdw1==1&&ggdw2==1]
    on18 -> songkaishijian6
    (junction 410) -> on18 [order 1] : [yjt>2]
  (default) -> zidong
  data: start input; kgdw1 input; kgdw2 input; skhx output; kghx output; kgzhiling1 output; kgzhiling2 output; yjhx output; gghx output; ggzhiling1 output; ggzhiling2 output; skt output; kgt output; sdt output; jst output; ggt output; yjt output; ggdw1 input; ggdw2 input; kghc input; gghc input; sddw input; yjdw input; skdw input; jsdw input; t1 input; t3 input; t5 input; t7 input; t9 input; t11 input; t local; t2 local; t4 local; t6 local; t8 local; shedingcishu input; yikaicishu output; skyichang output; kgyichang output; sdyichang output; jsyichang output; jieshu input; t10 local; ggyichang output; yjyichang output

== stateflow chart aaa/Subsystem1/shoudong/Chart1 ==
  state off
    en:
    skhx=0;
    kghx=0;
    gghx=0;
    yjhx=0;
    kgzhiling1=0;
    kgzhiling2=0;
    ggzhiling1=0;
    ggzhiling2=0;
    skyichang=0;
    kgyichang=0;
    sdyichang=0;
    jsyichang=0;
    ggyichang=0;
    yjyichang=0;
  state shoudong
    state songkai [parallel]
      settings: executionOrder=1
      state off
        entry:
        skhx=0;
        skt=0;
      state on
        entry:
        skhx=1;
        skyichang=0;
      state t
        entry:
        skt=skt+0.002;
      state t1
        entry:
        skyichang=1;
      state t2
        entry:
        skt=skt+0.002;
      (default) -> shoudong.songkai.off
      shoudong.songkai.t2 -> shoudong.songkai.off [order 2] : [skdw==1&&jsdw==1&&songkai==0]
      (junction 19) -> shoudong.songkai.off [order 2] : [skdw==1&&jsdw==1&&songkai==0]
      shoudong.songkai.off -> shoudong.songkai.on : [songkai==1&&yjdw==1&&sddw==1]
      shoudong.songkai.on -> (junction 19)
      shoudong.songkai.t -> (junction 19) : after(1,tick)
      (junction 19) -> shoudong.songkai.t1 [order 3] : [skt>2]
      (junction 19) -> shoudong.songkai.t [order 1] : [skdw==0]
      shoudong.songkai.t1 -> shoudong.songkai.t2
      shoudong.songkai.t2 -> shoudong.songkai.t2 [order 1] : [skdw==0]
    state kaigai [parallel]
      settings: executionOrder=2
      state off
        entry:
        kghx=0;
        kgt=0;
        kgzhiling1=0;
        kgzhiling2=0
      state on
        entry:
        kghx=1;
        kgzhiling1=1;
        kgzhiling2=1;
        kgyichang=0;
      state t
        entry:
        kgt=kgt+1;
      state t1
        entry:
        kgyichang=1;
      state t2
        entry:
        kgt=kgt+0.002;
      (default) -> shoudong.kaigai.off
      shoudong.kaigai.t2 -> shoudong.kaigai.off [order 2] : [kgdw1==1&&kgdw2==1&&kaigai==0]
      (junction 39) -> shoudong.kaigai.off [order 2] : [kgdw1==1&&kgdw2==1&&kaigai==0]
      shoudong.kaigai.off -> shoudong.kaigai.on : [kaigai==1&&skdw==1&&jsdw==1]
      shoudong.kaigai.on -> (junction 39)
      (junction 39) -> shoudong.kaigai.t1 [order 3] : [kgt>12]
      shoudong.kaigai.t -> (junction 39) : after(1,tick)
      (junction 39) -> shoudong.kaigai.t [order 1] : [kgdw1==0&&kgdw2==0]
      shoudong.kaigai.t1 -> shoudong.kaigai.t2
      shoudong.kaigai.t2 -> shoudong.kaigai.t2 [order 1] : [kgdw1==0&&kgdw2==0]
    state jiesuo [parallel]
      settings: executionOrder=4
      state off
        entry:
        skhx=0;
        jst=0;
      state on
        entry:
        skhx=1;
        jsyichang=0;
      state t
        entry:
        jst=jst+1;
      state t1
        entry:
        jsyichang=1;
      state t2
        entry:
        jst=jst+0.002;
      (default) -> shoudong.jiesuo.off
      shoudong.jiesuo.t2 -> shoudong.jiesuo.off [order 2] : [jsdw==1&&skdw==1&&jiesuo==0]
      (junction 60) -> shoudong.jiesuo.off [order 2] : [jsdw==1&&skdw==1&&jiesuo==0]
      shoudong.jiesuo.off -> shoudong.jiesuo.on : [jiesuo==1&&yjdw==1&&sddw==1&&kgdw1==1&&kgdw2==1]
      shoudong.jiesuo.on -> (junction 60)
      (junction 60) -> shoudong.jiesuo.t1 [order 3] : [sdt>2]
      shoudong.jiesuo.t -> (junction 60) : after(1,tick)
      (junction 60) -> shoudong.jiesuo.t [order 1] : [jsdw==0&&skdw==0]
      shoudong.jiesuo.t1 -> shoudong.jiesuo.t2
      shoudong.jiesuo.t2 -> shoudong.jiesuo.t2 [order 1] : [jsdw==0&&skdw==0]
    state suoding [parallel]
      settings: executionOrder=3
      state off
        entry:
        yjhx=0;
        sdt=0;
      state on
        entry:
        yjhx=1;
        sdyichang=0;
      state t1
        entry:
        sdyichang=1;
      state t2
        entry:
        sdt=sdt+0.002;
      state t
        entry:
        sdt=sdt+1;
      (default) -> shoudong.suoding.off
      shoudong.suoding.t2 -> shoudong.suoding.off [order 2] : [sddw==1&&yjdw==1&&suoding==0]
      (junction 48) -> shoudong.suoding.off [order 2] : [sddw==1&&yjdw==1&&suoding==0]
      shoudong.suoding.off -> shoudong.suoding.on : [suoding==1&&skdw==1&&jsdw==1&&kgdw1==1&&kgdw2==1]
      shoudong.suoding.on -> (junction 48)
      (junction 48) -> shoudong.suoding.t1 [order 3] : [sdt>2]
      shoudong.suoding.t -> (junction 48) : after(1,tick)
      (junction 48) -> shoudong.suoding.t [order 1] : [sddw==0&&yjdw==0]
      shoudong.suoding.t1 -> shoudong.suoding.t2
      shoudong.suoding.t2 -> shoudong.suoding.t2 [order 1] : [sddw==0&&yjdw==0]
    state yajin [parallel]
      settings: executionOrder=6
      state off
        entry:
        yjhx=0;
        yjt=0;
      state on
        entry:
        yjhx=1;
        yjyichang=0;
      state t3
        entry:
        yjyichang=1;
      state t2
        entry:
        sdt=sdt+0.002;
      state t
        entry:
        yjt=yjt+1;
      (default) -> shoudong.yajin.off
      shoudong.yajin.t2 -> shoudong.yajin.off [order 2] : [yjdw==1&&sddw==1&&yajin==0]
      (junction 94) -> shoudong.yajin.off [order 2] : [yjdw==1&&sddw==1&&yajin==0]
      shoudong.yajin.off -> shoudong.yajin.on : [yajin==1&&ggdw1==1&&ggdw2==1&&jsdw==1&&skdw==1]
      shoudong.yajin.on -> (junction 94)
      (junction 94) -> t3 [order 3] : [ggt>12]
      shoudong.yajin.t -> (junction 94) : after(1,tick)
      (junction 94) -> shoudong.yajin.t [order 1] : [yjdw==0&&sddw==0]
      t3 -> shoudong.yajin.t2
      shoudong.yajin.t2 -> shoudong.yajin.t2 [order 1] : [yjdw==0&&sddw==0]
    state guangai [parallel]
      settings: executionOrder=5
      state off
        entry:
        gghx=0;
        ggt=0;
        ggzhiling1=0;
        ggzhiling2=0
      state on
        entry:
        gghx=1;
        ggzhiling1=1;
        ggzhiling2=1;
        ggyichang=0;
      state t1
        entry:
        ggyichang=1;
      state t2
        entry:
        sdt=sdt+0.002;
      state t
        entry:
        ggt=ggt+1;
      (default) -> shoudong.guangai.off
      shoudong.guangai.t2 -> shoudong.guangai.off [order 2] : [ggdw1==1&&ggdw2==1&&guangai==0]
      (junction 81) -> shoudong.guangai.off [order 2] : [ggdw1==1&&ggdw2==1&&guangai==0]
      shoudong.guangai.off -> shoudong.guangai.on : [guangai==1&&skdw==1&&jsdw==1]
      shoudong.guangai.on -> (junction 81)
      (junction 81) -> shoudong.guangai.t1 [order 3] : [ggt>12]
      shoudong.guangai.t -> (junction 81) : after(1,tick)
      (junction 81) -> shoudong.guangai.t [order 1] : [ggdw1==0&&ggdw2==0]
      shoudong.guangai.t1 -> shoudong.guangai.t2
      shoudong.guangai.t2 -> shoudong.guangai.t2 [order 1] : [ggdw1==0&&ggdw2==0]
  state off1
    en:
    skhx=0;
    kghx=0;
    gghx=0;
    yjhx=0;
    kgzhiling1=0;
    kgzhiling2=0;
    ggzhiling1=0;
    ggzhiling2=0;
  (default) -> off
  off -> shoudong : [start==1&&jieshu==0]
  shoudong -> off1 : [jieshu==1]
  data: start input; kgdw1 input; kgdw2 input; ggdw1 input; ggdw2 input; sddw input; jsdw input; yjdw input; skdw input; songkai input; kaigai input; suoding input; jiesuo input; skhx output; kghx output; yjhx output; gghx output; kgzhiling1 output; kgzhiling2 output; ggzhiling1 output; ggzhiling2 output; skt output; kgt output; sdt output; jst output; ggt output; guangai input; yajin input; yjt output; skyichang output; kgyichang output; sdyichang output; jsyichang output; jieshu input; ggyichang output; yjyichang output
